simulink library "rpsrootlib"  (R2013b)
settings: Solver=ode45  StartTime=0.0  StopTime=10.0  RelTol=1e-3
settings Model: Creator=Q365198  LastModifiedBy=Q365198

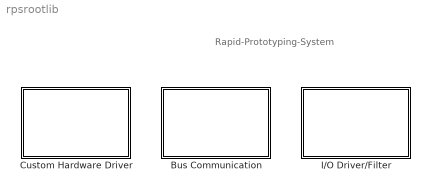
== system rpsrootlib ==
  note: Rapid-Prototyping-System
  Bus Communication : Subsystem
      mask Display: fprintf('Communication')
  Custom Hardware Driver : Subsystem
      mask Display: fprintf('Driver')
  I/O Driver/Filter : Subsystem
      mask Display: fprintf('I/O')

== system rpsrootlib/Bus Communication ==

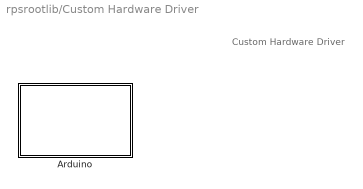
== system rpsrootlib/Custom Hardware Driver ==
  note: Custom Hardware Driver
  Arduino : Subsystem
      mask Display: fprintf('Custom Arduino')

== system rpsrootlib/I//O Driver//Filter ==

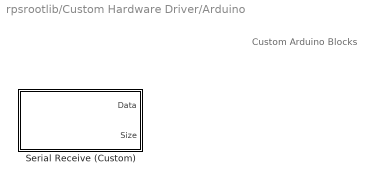
== system rpsrootlib/Custom Hardware Driver/Arduino ==
  note: Custom Arduino Blocks
  Serial Receive (Custom) : Subsystem  mask(Arduino Serial Receive (Custom)){bufferSize=64, comPort=0, SampleTime=-1}
      mask prompts: bufferSize "Receive Buffer Size (1 - 64 Bytes):"; comPort "Port number:"; SampleTime "Sample Time (-1 for inherited)"
      mask help:
      | Get bytes of data from the specified serial port and write it to the Data block output. Maximum Datasize can be defined (64 Bytes = Hardware Buffer).
      |
      | If data is received, Status block output gives the size of the received data. If data is not received, Status is equal 0.
      |
      | Enter the number of the serial port (0 for Arduino Uno, 0-3 for Arduino Mega 2560). Do not assign the same port to more than one Serial Receive block.
      |
      | Serial ports use the following digital pins:
      | - Port 0: pin 0
      | - Port 1: pin 19
      | - Port 2: pin 17
      | - Port 3: pin 15
      mask Display:
      | pic=imread('serial.png');image(pic,[0.28 0.18 0.45 0.65]);text(0.5, 0.15, 'Port 0', 'horizontalAlignment', 'center');
      | color('blue');
      | text(0.55, 0.87, 'ARDUINO', 'horizontalAlignment', 'left');
      | color('black');
      | port_label('output', 1, 'Data');
      | port_label('output', 2, 'Status');

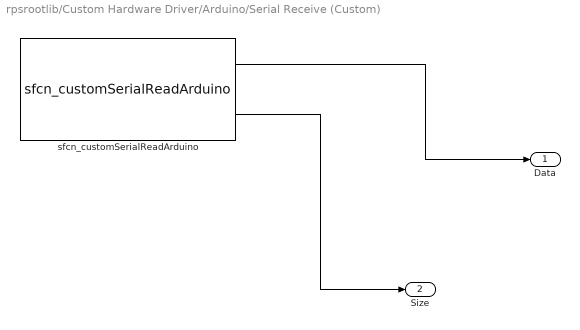
== system rpsrootlib/Custom Hardware Driver/Arduino/Serial Receive (Custom) ==
  sfcn_customSerialReadArduino : S-Function  FunctionName=sfcn_customSerialReadArduino  Parameters=comPort, bufferSize, SampleTime  EnableBusSupport=off  mask(Legacy Function){SFunctionSpec=customSerial_Read(int32 p1, uint8 y1[p2], int32 y2[1], int32 p2), ShowSpec=on}
      mask prompts: ShowSpec "Display function specification"
      mask help:
      | This block allows you to call the legacy functions specified by the following Legacy Code Tool definition:
      | def.SFunctionName = 'sfcn_customSerialReadArduino';
      | def.OutputFcnSpec = 'customSerial_Read(int32 p1, uint8 y1[p2], int32 y2[1], int32 p2)';
      | def.HeaderFiles = {'customArduino.h'};
      | def.SourceFiles = {'customArduino.c'};
      | def.IncPaths = {'C:\Users\q365198\Rapid-Prototyping-System\blocks\src\customArduino\'};
      | def.SrcPaths = {'C:\Users\q365198\Rapid-Prototyping-System\blocks\src\customArduino\'};
      | def.SampleTime = 'parameterized';
      mask Help: <p>This block was generated automatically by the Legacy Code Tool. For detailed help on this tool, call<a href="matlab:legacy_code('help')"> legacy_code('help')</a>.</p>
      mask Callback ShowSpec:
      | if strcmp(get_param(gcbh, 'ShowSpec'), 'on')
      |   set_param(gcbh, 'MaskDisplay', sprintf('fprintf(''%s'');', get_param(gcbh, 'SFunctionSpec')));
      | else
      |   set_param(gcbh, 'MaskDisplay', sprintf('fprintf(''%s'');', get_param(gcbh, 'FunctionName')));
      | end
      mask Display: fprintf('customSerial_Read(int32 p1, uint8 y1[p2], int32 y2[1], int32 p2)');
  Data : Outport
  Size : Outport  Port=2
  wires:
  sfcn_customSerialReadArduino/2 -> Size/1
  sfcn_customSerialReadArduino/1 -> Data/1
